simulink model "ArduinoController"  (R2020a)
settings: Solver=FixedStepAuto  StartTime=0.0  StopTime=30  FixedStep=Ts  MaxStep=0.015  RelTol=1e-3
PreLoadFcn:
  | if ~exist('sim_HIL')
  |     sim_HIL=false;
  | end
  | if ~exist('usefilter')
  |     usefilter=false;
  | end
InitFcn:
  | load motorModel.mat
  | load expsetup
model workspace (MAT data in the model file):
  C = [5001.86332222 94.647196767]
  N = 10
  Ts = 0.015
  del = 0.938968768187
  delt = 0.938968768187
  dsys = idss
  dsys.InputName_ = "Time"
  dsys.InputUnit_ = "s"
  dsys.OutputName_ = ["Position"; "Velocity"]
  dsys.OutputUnit_ = ["rad"; "rad/s"]
  dsys.IOSize_ = [2 1]
  dsys.Data_ = idpack.ssdata
  dsys.Data_.X0 = param.Continuous
  dsys.Data_.X0.Free_ = [0; 0]
  dsys.Data_.X0.Size_ = [2 1]
  dsys.Data_.X0.Value_ = [0; 0]
  dsys.Data_.X0.pID = paramid.Variable
  dsys.Data_.X0.pID.Name = 'x0'
  dsys.Data_.Structure = pmodel.ss
  dsys.Data_.Structure.A = param.Continuous
  dsys.Data_.Structure.A.Size_ = [2 2]
  dsys.Data_.Structure.A.Value_ = [0.998217929097  0.0355618485158; 0.044388098097  0.00279539919437]
  dsys.Data_.Structure.A.pID = paramid.Variable
  dsys.Data_.Structure.A.pID.Name = 'A'
  dsys.Data_.Structure.B = param.Continuous
  dsys.Data_.Structure.B.Size_ = [2 1]
  dsys.Data_.Structure.B.Value_ = [0.00813093166564; 0.988691747082]
  dsys.Data_.Structure.B.pID = paramid.Variable
  dsys.Data_.Structure.B.pID.Name = 'B'
  dsys.Data_.Structure.C = param.Continuous
  dsys.Data_.Structure.C.Size_ = [2 2]
  dsys.Data_.Structure.C.Value_ = [1  0; 0  1]
  dsys.Data_.Structure.C.pID = paramid.Variable
  dsys.Data_.Structure.C.pID.Name = 'C'
  dsys.Data_.Structure.D = param.Continuous
  dsys.Data_.Structure.D.Free_ = [0; 0]
  dsys.Data_.Structure.D.Size_ = [2 1]
  dsys.Data_.Structure.D.Value_ = [0; 0]
  dsys.Data_.Structure.D.pID = paramid.Variable
  dsys.Data_.Structure.D.pID.Name = 'D'
  dsys.Data_.Structure.K = param.Continuous
  dsys.Data_.Structure.K.Free_ = [0  0; 0  0]
  dsys.Data_.Structure.K.Size_ = [2 2]
  dsys.Data_.Structure.K.Value_ = [0  0; 0  0]
  dsys.Data_.Structure.K.pID = paramid.Variable
  dsys.Data_.Structure.K.pID.Name = 'K'
  dsys.Data_.NoiseVariance = [0.154630276497  0.617377315059; 0.617377315059  6.29681093335]
  dsys.Data_.InterSample = {'zoh'}
  dsys.Data_.Report = idresults.ssest
  dsys.Data_.Report.Fit.FitPercent = []
  dsys.Data_.Report.Fit.LossFcn = []
  dsys.Data_.Report.Fit.MSE = []
  dsys.Data_.Report.Fit.FPE = []
  dsys.Data_.Report.Fit.AIC = []
  dsys.Data_.Report.Fit.AICc = []
  dsys.Data_.Report.Fit.nAIC = []
  dsys.Data_.Report.Fit.BIC = []
  dsys.Data_.Report.Parameters.ParVector = []
  dsys.Data_.Report.Parameters.Free = []
  dsys.Data_.Report.Parameters.Labels = {}
  dsys.Data_.Report.Parameters.FreeParCovariance = []
  dsys.Data_.Report.Parameters.X0 = []
  dsys.Data_.Report.Parameters.X0Covariance = []
  dsys.Data_.Report.DataUsed.Name = ''
  dsys.Data_.Report.DataUsed.Type = ''
  dsys.Data_.Report.DataUsed.Length = []
  dsys.Data_.Report.DataUsed.Ts = []
  dsys.Data_.Report.DataUsed.InterSample = ''
  dsys.Data_.Report.DataUsed.InputOffset = []
  dsys.Data_.Report.DataUsed.OutputOffset = []
  dsys.Data_.EstimationStatus = -Inf
  dsys.Data_.Delay.Input = 0
  dsys.Data_.Delay.Output = [0; 0]
  dsys.Data_.Ts = 0.015
  eta = 1
  gamm = 10.0000520274
  nodeID = 1
  qT = 1e-05
  vphi = 1.000013195
  xiT = 1e-05
libraries: simulink x1
settings Model: DataDictionary=MotorInfo.sldd  Creator=khoi  LastModifiedBy=khoi
settings DataIOCC: SaveOutput=off  SaveTime=off
settings OptimizationCC: DefaultParameterBehavior=Inlined  UseDivisionForNetSlopeComputation=on  GainParamInheritBuiltInType=on  UseFloatMulNetSlope=on  InlineInvariantSignals=on  PassReuseOutputArgsAs=Individual arguments  ZeroExternalMemoryAtStartup=off  ZeroInternalMemoryAtStartup=off  NoFixptDivByZeroProtection=on  EfficientFloat2IntCast=on  LifeSpan=1  OptimizeBlockOrder=speed  DifferentSizesBufferReuse=on  EfficientTunableParamExpr=on
settings DebuggingCC: ParameterTunabilityLossMsg=error
settings HardwareCC: ProdBitPerInt=16  ProdBitPerPointer=16  ProdBitPerSizeT=16  ProdBitPerPtrDiffT=16  ProdLargestAtomicFloat=None  ProdWordSize=8  ProdLongLongMode=on  ProdHWDeviceType=Atmel->AVR
settings SFSimCC: MATLABDynamicMemAlloc=off
settings RTWCC: SystemTargetFile=ert.tlc  TemplateMakefile=ert_default_tmf  GenerateReport=on  LaunchReport=on
settings CodeAppCC: ForceParamTrailComments=on  IgnoreCustomStorageClasses=off  OperatorAnnotations=on  SimulinkDataObjDesc=on  SFDataObjDesc=on  CustomSymbolStrGlobalVar=rt$N$M  CustomSymbolStrType=$N$M  CustomSymbolStrFcn=$N$M$F  CustomSymbolStrMacro=$N$M  InsertBlockDesc=on
settings ERTTargetCC: TargetLangStandard=C99 (ISO)  GenerateSampleERTMain=on  IncludeMdlTerminateFcn=off  CombineSignalStateStructs=on  SupportComplex=off  SupportContinuousTime=on  SupportNonInlinedSFcns=on  InlinedParameterPlacement=NonHierarchical  ERTCustomFileTemplate=example_file_process.tlc  ERTFilePackagingFormat=CompactWithDataFile

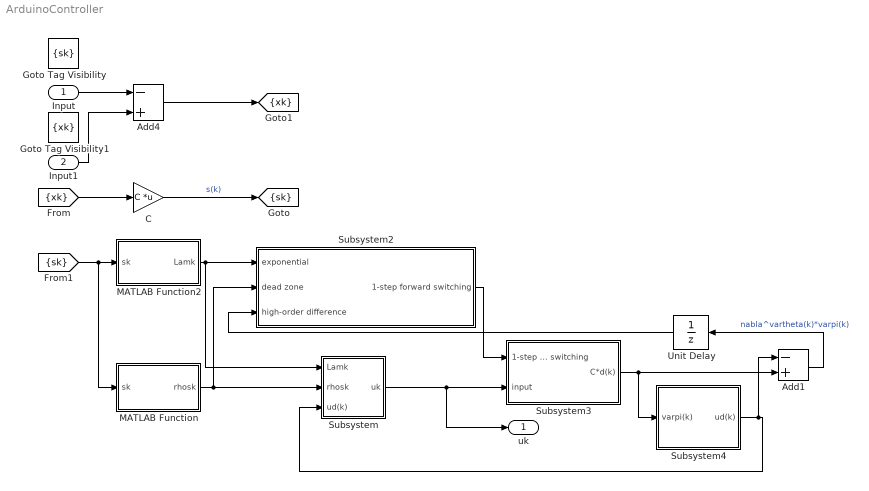
== system ArduinoController ==
  Input : Inport  PortDimensions=2
  Input1 : Inport  Port=2  PortDimensions=2
  Add1 : Sum  Inputs=-+
  Add4 : Sum  Inputs=-+
  C : Gain  Gain=C  Multiplication=Matrix(K*u) (u vector)
  Goto Tag Visibility : GotoTagVisibility  GotoTag=sk
  Goto Tag Visibility1 : GotoTagVisibility  GotoTag=xk
  MATLAB Function : MATLAB Function  TreatAsAtomicUnit=on  mask{eta=eta}
      mask prompts: eta "eta>0"
  MATLAB Function2 : MATLAB Function  TreatAsAtomicUnit=on  mask{del=delt, vphi=vphi, gam=round(gamm)}
      mask prompts: del "0<delta<1"; vphi "vphi>0"; gam "gamma>0 natrual number"
  Subsystem : Subsystem
  Subsystem2 : Subsystem
  Subsystem3 : Subsystem
  Subsystem4 : Subsystem
  Unit Delay : UnitDelay  SampleTime=-1  HasFrameUpgradeWarning=on
  uk : Outport  PortDimensions=1
  tag scope: sk=scoped, xk=scoped
  wires:
  Unit Delay/1 -> Subsystem2/3(high-order difference)
  [sk] -> MATLAB Function/1(sk), MATLAB Function2/1(sk)
  Add4/1 -> [xk]
  C/1 -> [sk]  "s(k)"
  [xk] -> C/1
  Input/1 -> Add4/1
  MATLAB Function/1(rhosk) -> Subsystem2/2(dead zone), Subsystem/2(rhosk)
  Input1/1 -> Add4/2
  Add1/1 -> Unit Delay/1  "nabla^vartheta(k)*varpi(k)"
  Subsystem2/1(1-step forward switching) -> Subsystem3/1(1-step forward switching)
  Subsystem/1(uk) -> Subsystem3/2(input), uk/1
  Subsystem4/1(ud(k)) -> Add1/1, Subsystem/3(ud(k))
  Subsystem3/1(C*d(k)) -> Subsystem4/1(varpi(k)), Add1/2
  MATLAB Function2/1(Lamk) -> Subsystem2/1(exponential), Subsystem/1(Lamk)

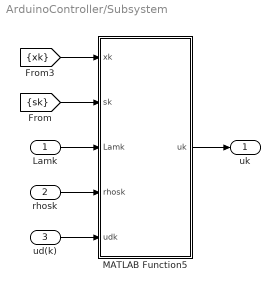
== system ArduinoController/Subsystem ==
  Lamk : Inport
  rhosk : Inport  Port=2
  ud(k) : Inport  Port=3
  MATLAB Function5 : MATLAB Function  TreatAsAtomicUnit=on  mask{Phi=dsys.A, Gam=dsys.B, C=C, qT=qT, xiT=xiT}
  uk : Outport
  wires:
  [xk] -> MATLAB Function5/1(xk)
  ud(k)/1 -> MATLAB Function5/5(udk)
  MATLAB Function5/1(uk) -> uk/1
  Lamk/1 -> MATLAB Function5/3(Lamk)
  rhosk/1 -> MATLAB Function5/4(rhosk)
  [sk] -> MATLAB Function5/2(sk)

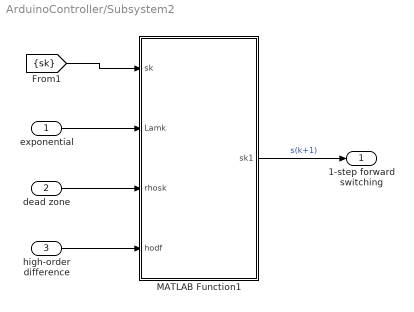
== system ArduinoController/Subsystem2 ==
  exponential : Inport
  dead zone : Inport  Port=2
  high-order difference : Inport  Port=3
  MATLAB Function1 : MATLAB Function  TreatAsAtomicUnit=on  mask{xiT=xiT, qT=qT}
      mask prompts: xiT "xi > 0 (xiT>0)"; qT "q (0<1-qT<1)"
  1-step forward switching : Outport
  wires:
  [sk] -> MATLAB Function1/1(sk)
  MATLAB Function1/1(sk1) -> 1-step forward switching/1  "s(k+1)"
  high-order difference/1 -> MATLAB Function1/4(hodf)
  dead zone/1 -> MATLAB Function1/3(rhosk)
  exponential/1 -> MATLAB Function1/2(Lamk)

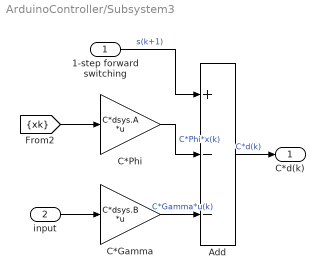
== system ArduinoController/Subsystem3 ==
  1-step forward switching : Inport
  input : Inport  Port=2
  Add : Sum  Inputs=+--
  C*Gamma : Gain  Gain=C*dsys.B  Multiplication=Matrix(K*u)
  C*Phi : Gain  Gain=C*dsys.A  Multiplication=Matrix(K*u) (u vector)
  C*d(k) : Outport
  wires:
  C*Gamma/1 -> Add/3  "C*Gamma*u(k)"
  C*Phi/1 -> Add/2  "C*Phi*x(k)"
  input/1 -> C*Gamma/1
  Add/1 -> C*d(k)/1  "C*d(k)"
  [xk] -> C*Phi/1
  1-step forward switching/1 -> Add/1  "s(k+1)"

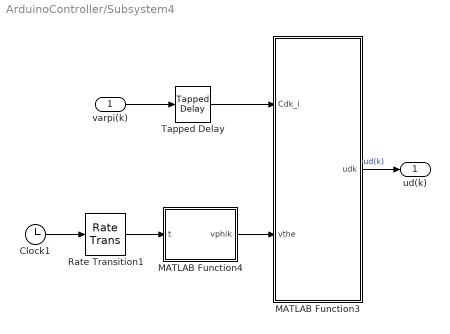
== system ArduinoController/Subsystem4 ==
  varpi(k) : Inport
  Clock1 : Clock
  MATLAB Function3 : MATLAB Function  TreatAsAtomicUnit=on
  MATLAB Function4 : MATLAB Function  TreatAsAtomicUnit=on  mask{Ts=Ts, n=round(N)}
  Rate Transition1 : RateTransition  OutPortSampleTime=Ts
  Tapped Delay : simulink/Discrete/Tapped Delay  vinit=0.0  samptime=-1  NumDelays=round(N)  DelayOrder=Newest  includeCurrent=off
  ud(k) : Outport
  wires:
  Tapped Delay/1 -> MATLAB Function3/1(Cdk_i)
  Clock1/1 -> Rate Transition1/1
  Rate Transition1/1 -> MATLAB Function4/1(t)
  MATLAB Function4/1(vphik) -> MATLAB Function3/2(vthe)
  varpi(k)/1 -> Tapped Delay/1
  MATLAB Function3/1(udk) -> ud(k)/1  "ud(k)"

== matlab function ArduinoController/MATLAB Function ==
  data: sk input; rhosk output; eta parameter
function rhosk = fDeadzone(sk,eta)
    if sk>eta
        rhosk=1;
    elseif abs(sk)<=eta
        rhosk=0;
    else % sk<-eta
        rhosk=-1;
    end

== matlab function ArduinoController/MATLAB Function2 ==
  data: sk input; Lamk output; del parameter; vphi parameter; gam parameter
function Lamk = fLambda(sk,del,vphi,gam)
Lamk= del + (1-del)*exp(-vphi*abs(sk)^gam);

== matlab function ArduinoController/Subsystem/MATLAB Function5 ==
  data: xk input; uk output; sk input; Lamk input; rhosk input; udk input; Phi parameter; Gam parameter; C parameter; qT parameter; xiT parameter
function uk = fcn(xk,sk,Lamk,rhosk,udk,...
    Phi, Gam, C, qT, xiT)

uk = -(C*Gam)\(C*Phi*xk - (1-qT)*Lamk*sk + xiT/Lamk*rhosk + udk);

== matlab function ArduinoController/Subsystem2/MATLAB Function1 ==
  data: sk input; sk1 output; Lamk input; rhosk input; hodf input; xiT parameter; qT parameter
function sk1 = fFwrdSwit(sk,Lamk,rhosk,hodf,...
    xiT, qT)

sk1 = (1-qT)*Lamk*sk - xiT/Lamk*rhosk + hodf;

== matlab function ArduinoController/Subsystem4/MATLAB Function3 ==
  data: Cdk_i input; vthe input; udk output
function udk = fDtbCompen(Cdk_i,vthe)
udk = 0;
for i=1:vthe
    udk = udk - (-1)^i*nchoosek(vthe,i)*Cdk_i(i);
end

== matlab function ArduinoController/Subsystem4/MATLAB Function4 ==
  data: t input; vphik output; Ts parameter; n parameter
function vphik = fVphi(t,Ts,n)
persistent k;
if isempty(k)
    k=0;
end
if rem(t,Ts)==0 && t~=0 && k<n
    k = k+1;
end
vphik = k;
